simulink model "milestoneone"  (R2025a)
settings: Solver=FixedStepAuto  StartTime=0.0  StopTime=10  FixedStep=1e-3  RelTol=1e-3  EnableMultiTasking=on
model workspace (MAT data in the model file):
  Var = 0
settings Model: ExtModeTrigDuration=5  Creator=alber  LastModifiedBy=alber
settings OptimizationCC: DefaultParameterBehavior=Inlined  EnhancedBackFolding=on  PassReuseOutputArgsAs=Individual arguments  ZeroExternalMemoryAtStartup=off  ZeroInternalMemoryAtStartup=off  MaxStackSize=64  OptimizeBlockOrder=speed  DifferentSizesBufferReuse=on  OptimizationCustomize=off  EfficientTunableParamExpr=on
settings DebuggingCC: ParameterTunabilityLossMsg=error
settings HardwareCC: ProdBitPerPointer=32.0  ProdBitPerSizeT=32.0  ProdBitPerPtrDiffT=32.0  ProdLargestAtomicInteger=Long  ProdLargestAtomicFloat=Double  ProdWordSize=32.0  ProdHWDeviceType=ARM Compatible->ARM Cortex
settings SFSimCC: MATLABDynamicMemAlloc=off
settings RTWCC: SystemTargetFile=ert.tlc  HardwareBoard=NXP FRDM-K64F  TLCOptions="-aInlineSetEventsForThisBaseRateFcn=TLC_FALSE -aSuppressMultiTaskScheduler=TLC_FALSE  -aRateBasedStepFcn=0"  TemplateMakefile=ert_default_tmf  Toolchain=GNU Tools for ARM Embedded Processors  Description=Embedded Coder
settings CodeAppCC: ForceParamTrailComments=on  IgnoreCustomStorageClasses=off  OperatorAnnotations=on  SimulinkDataObjDesc=on  SFDataObjDesc=on  InsertBlockDesc=on
settings ERTTargetCC: ExtModeTransport=4.0  ExtModeStaticAlloc=off  ExtModeMexFile=sendToCommService  ExtModeIntrfLevel=Level1

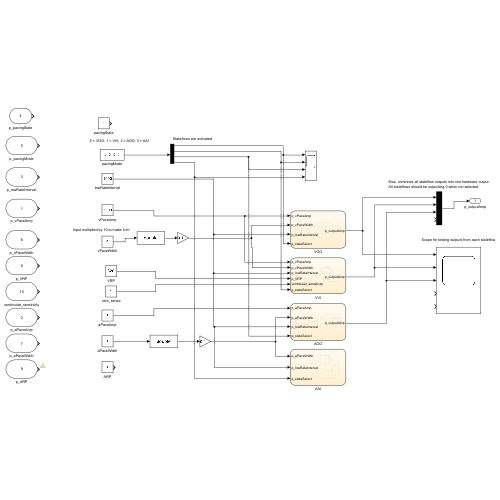
[thumbnail: Simulink's stored preview of the top-level diagram]
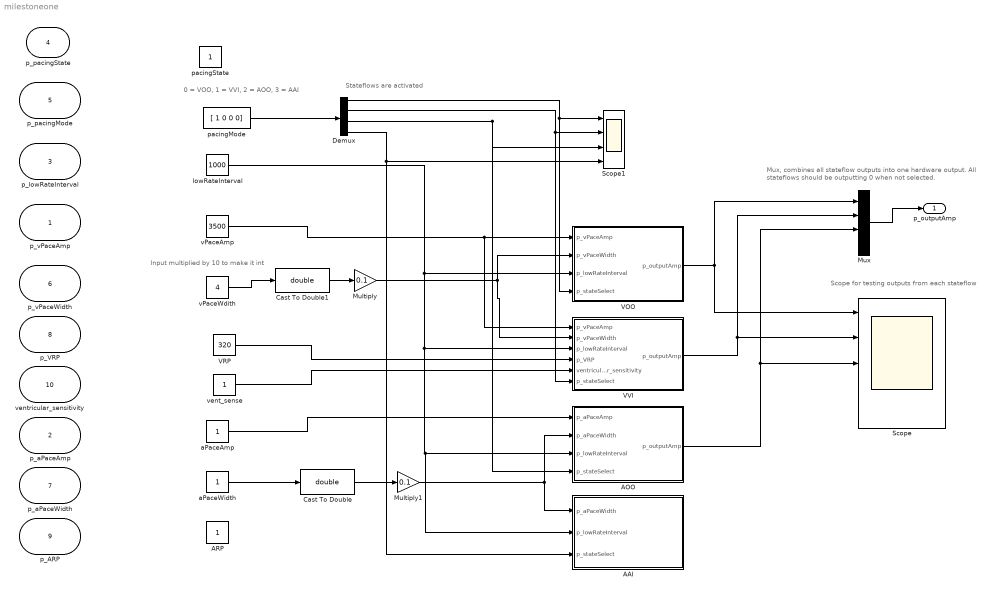
== system milestoneone ==
  note: Stateflows are activated
  note: Input multiplied by 10 to make it int
  note: 0 = VOO, 1 = VVI, 2 = AOO, 3 = AAI
  note: Scope for testing outputs from each stateflow
  note: Mux, combines all stateflow outputs into one hardware output.
      | All stateflows should be outputting 0 when not selected.
  p_vPaceAmp : Inport  OutMin=[500]  OutMax=[7000]  OutDataTypeStr=uint16  Unit=mV  PortDimensions=1
  p_aPaceAmp : Inport  Port=2  OutDataTypeStr=uint16  Unit=mV  PortDimensions=1
  p_lowRateInterval : Inport  Port=3  OutMin=[343]  OutMax=[2000]  OutDataTypeStr=uint16  Unit=Msec  PortDimensions=1
  p_pacingState : Inport  Port=4
  p_pacingMode : Inport  Port=5  OutDataTypeStr=uint8  PortDimensions=1
  p_vPaceWidth : Inport  Port=6  OutMin=1  OutMax=1.9  OutDataTypeStr=uint16  Unit=Msec  PortDimensions=1
  p_aPaceWidth : Inport  Port=7  OutDataTypeStr=uint16  Unit=Msec  PortDimensions=1
  p_VRP : Inport  Port=8  OutMin=[150]  OutMax=[500]  OutDataTypeStr=uint16  Unit=Msec  PortDimensions=1
  p_ARP : Inport  Port=9  OutDataTypeStr=uint16  Unit=mSec  PortDimensions=1
  ventricular_sensitivity : Inport  Port=10  OutDataTypeStr=uint16  PortDimensions=1
  AAI : Stateflow chart  TreatAsAtomicUnit=on
  AOO : Stateflow chart  TreatAsAtomicUnit=on
  ARP : Constant  OutDataTypeStr=uint8
  Cast To Double : DataTypeConversion  OutDataTypeStr=double  SaturateOnIntegerOverflow=off  RndMeth=Floor
  Cast To Double1 : DataTypeConversion  OutDataTypeStr=double  SaturateOnIntegerOverflow=off  RndMeth=Floor
  Demux : Demux
  Multiply : Gain  Gain=0.1
  Multiply1 : Gain  Gain=0.1
  Mux : Mux
  Scope : Scope  NumInputPorts=5
      settings: ActiveDisplayYMinimum=-2035.2732414864563  ActiveDisplayYMaximum=4435.8066355354867
  Scope1 : Scope  NumInputPorts=4
      settings: ActiveDisplayYMinimum=-0.21829770302879026  ActiveDisplayYMaximum=1.817820580443013
  VOO : Stateflow chart  TreatAsAtomicUnit=on
  VRP : Constant  Value=320  OutMin=[150]  OutMax=[500]  OutDataTypeStr=uint16
  VVI : Stateflow chart  TreatAsAtomicUnit=on
  aPaceAmp : Constant  OutDataTypeStr=uint16
  aPaceWidth : Constant  OutDataTypeStr=int16
  lowRateInterval : Constant  Value=1000  OutMin=[343]  OutMax=[2000]  OutDataTypeStr=uint16
  pacingMode : Constant  Value=[ 1 0 0 0]  OutDataTypeStr=uint8
  pacingState : Constant  OutDataTypeStr=uint8
  vPaceAmp : Constant  Value=3500  OutMin=[500]  OutMax=[7000]  OutDataTypeStr=uint16
  vPaceWdith : Constant  Value=4  OutMin=[1]  OutMax=[19]  OutDataTypeStr=int16
  vent_sense : Constant  OutDataTypeStr=uint16
  p_outputAmp : Outport
  wires:
  VVI/1(p_outputAmp) -> Mux/2, Scope/2
  AOO/1(p_outputAmp) -> Mux/3, Scope/3
  Mux/1 -> p_outputAmp/1
  Multiply/1 -> VOO/2(p_vPaceWidth), VVI/2(p_vPaceWidth)
  Cast To Double1/1 -> Multiply/1
  Cast To Double/1 -> Multiply1/1
  Multiply1/1 -> AAI/1(p_aPaceWidth), AOO/2(p_aPaceWidth)
  Demux/1 -> Scope1/1, VOO/4(p_stateSelect)
  Demux/2 -> Scope1/2, VVI/6(p_stateSelect)
  Demux/3 -> Scope1/3, AOO/4(p_stateSelect)
  Demux/4 -> AAI/3(p_stateSelect), Scope1/4
  pacingMode/1 -> Demux/1
  aPaceWidth/1 -> Cast To Double/1
  aPaceAmp/1 -> AOO/1(p_aPaceAmp)
  lowRateInterval/1 -> AAI/2(p_lowRateInterval), AOO/3(p_lowRateInterval), VVI/3(p_lowRateInterval), VOO/3(p_lowRateInterval)
  vPaceAmp/1 -> VVI/1(p_vPaceAmp), VOO/1(p_vPaceAmp)
  vPaceWdith/1 -> Cast To Double1/1
  VRP/1 -> VVI/4(p_VRP)
  vent_sense/1 -> VVI/5(ventricular_sensitivity)
  VOO/1(p_outputAmp) -> Scope/1, Mux/1

== stateflow chart milestoneone/VOO ==
  state CHARGE
    entry:
    % Output 0V
    p_outputAmp = 0;
    current_state = "VOO CHARGE"
    % Rest time = total cycle time - pace width
  state PACE
    entry:
    % Output pace at specified amplitude
    p_outputAmp = p_vPaceAmp;
    current_state = "VOO PACE"
    % Wait so that the pace has the specified width
  state INACTIVE
  CHARGE -> PACE [order 2] : [after(p_lowRateInterval - p_vPaceWidth, msec)]
  (default) -> INACTIVE
  INACTIVE -> CHARGE [order 1] : [p_stateSelect == 1]
  CHARGE -> INACTIVE [order 1] : [p_stateSelect == 0]
  INACTIVE -> INACTIVE [order 2] : [p_stateSelect == 0]
  PACE -> CHARGE : after(p_vPaceWidth, msec)
  data: data local; p_outputAmp output uint16; p_vPaceAmp input uint16 =3500; p_vPaceWidth input double =0.4; p_lowRateInterval input uint16 =6000/low_rate_lim; p_stateSelect input uint8; current_state local string

== stateflow chart milestoneone/AAI ==
  state PACING
    entry:
    state_out = "AAI PACING"
    AP = true; % deliver pacing pulse
    In_ARP = false;
    timer = 0;
    during:
    timer = timer + 1;
    if (timer >= p_aPaceWidth)
    % Pulse width elapsed -> stop pacing
    AP = false;
    % -> Refractory
    end
  state WAIT
    entry:
    state_out = "AAI WAIT";
    AP = false;
    In_ARP = false;
    timer = 0;
    during:
    if (AS && ~In_ARP)
    % Detected intrinsic atrial beat before timeout
    timer = 0;
    %transition_to(Refractory);
    % ^ Causes an error, add back in later
    elseif (timer >= p_lowRateInterval)
    %Timeout -> no intrinsic beat, deliver pulse
    % ->Pacing
    end
  state INACTIVE
  state Refractory
    entry:
    state_out = "AAI REFRACTORY"
    In_ARP = true;
    AP = false;
    timer = 0;
    during:
    timer = timer + 1;
    % Ignore all AS during ARP
    if (timer >= ARP)
    In_ARP = false;
    timer = 0;
    % -> Waiting
    end
  WAIT -> PACING [order 2] : [timer >= p_lowRateInterval]
  PACING -> Refractory : [after(p_aPaceWidth, msec)]
  (default) -> INACTIVE
  INACTIVE -> WAIT [order 1] : [p_stateSelect == 1]
  WAIT -> INACTIVE [order 1] : [p_stateSelect == 0]
  INACTIVE -> INACTIVE [order 2] : [p_stateSelect == 0]
  WAIT -> Refractory [order 3] : [AS && In_ARP]
  Refractory -> WAIT : [after(ARP, msec)]
  data: data local; data local; p_aPaceWidth input double =0.4; p_lowRateInterval input uint16 =6000/low_rate_lim; AP local boolean =false; In_ARP local boolean =false; ARP local uint16 =0; AS local uint16 =0; timer local uint16 =0; p_stateSelect input; state_out local string

== stateflow chart milestoneone/VVI ==
  state PACING
    entry:
    %current_state = "VVI PACING"
    output_pulse_flag = 0;
    p_outputAmp = 0;
    pacing_done_flag = 0;
  state WAIT
    entry:
    current_state = "VVI WAIT"
    output_pulse_flag = 0;
    p_outputAmp = 0;
    during:
    if (p_vPaceAmp == ventricular_sensitivity)
    output_pulse_flag = 1;
    p_outputAmp = p_vPaceAmp;
    end
  state REFRACTORY
    entry:
    current_state = "VVI REFRACTORY"
    output_pulse_flag = 1;
    p_outputAmp = p_vPaceAmp;
  state INACTIVE
    % When stateflow isn't selected
  PACING -> PACING [order 2] : after(p_vPaceWidth, msec){pacing_done_flag = 1;}
  PACING -> REFRACTORY [order 1] : [pacing_done_flag == 1]
  (default) -> INACTIVE
  WAIT -> PACING [order 3] : [after(p_lowRateInterval, msec) && (output_pulse_flag == 0)]
  INACTIVE -> WAIT [order 1] : [p_stateSelect == 1]
  REFRACTORY -> WAIT : [after(p_VRP, msec)]
  WAIT -> INACTIVE [order 1] : [p_stateSelect == 0]
  INACTIVE -> INACTIVE [order 2] : [p_stateSelect == 0]
  WAIT -> WAIT [order 2] : [after(p_lowRateInterval, msec) && (output_pulse_flag ==1)]
  data: p_vPaceAmp input uint16 =3500; p_vPaceWidth input double =0.4; p_lowRateInterval input uint16 =6000/low_rate_lim; output_pulse_flag local double; pacing_done_flag local double; p_VRP input uint16; ventricular_sensitivity input uint16; p_outputAmp output uint16; p_stateSelect input uint8; current_state local string

== stateflow chart milestoneone/AOO ==
  state PACE
    entry:
    output_pace_flag = true;
    p_outputAmp = p_aPaceAmp;
    current_state = "AOO PACE"
  state CHARGE
    entry:
    output_pace_flag = false;
    p_outputAmp = 0;
    current_state = "AOO CHARGE"
  state INACTIVE
    % When state is not selected by input
  CHARGE -> PACE [order 2] : [after(p_lowRateInterval - p_aPaceWidth, msec)]
  (default) -> INACTIVE
  INACTIVE -> CHARGE [order 1] : [p_stateSelect == 1]
  CHARGE -> INACTIVE [order 1] : [p_stateSelect == 0]
  INACTIVE -> INACTIVE [order 2] : [p_stateSelect == 0]
  PACE -> CHARGE : after(p_aPaceWidth, msec)
  data: data local; p_outputAmp output uint16; p_aPaceAmp input uint16 =3500; p_aPaceWidth input double =0.4; p_lowRateInterval input uint16 =6000/low_rate_lim; output_pace_flag local boolean; p_stateSelect input uint8; current_state local string
